simulink model "BMS_V4"  (R2017b)
settings: Solver=FixedStepDiscrete  StartTime=0.0  StopTime=inf  FixedStep=BASETIME  RelTol=1e-3  EnableMultiTasking=on
values from neighbouring files (symbols this model uses):
  AKT_BALANCE = uint16(8)    [BMS_V4_config.m]
  BALANCE = uint16(4)    [BMS_V4_config.m]
  BALANCE_RESISTOR = int32(5)    [BMS_V4_config.m]
  BALANCE_VEC = uint16(8)    [BMS_V4_config.m]
  CELL_SOC = uint16(7)    [BMS_V4_config.m]
  CELL_STATE = uint16(3)    [BMS_V4_config.m]
  CELL_TEMPERATURE = uint16(6)    [BMS_V4_config.m]
  CELL_VOLTAGE = uint16(5)    [BMS_V4_config.m]
  CELLACTBITFIELD = hex2dec('300')    [BMS_V4_config.m]
  CELLDEACTBITFIELD = hex2dec('100')    [BMS_V4_config.m]
  CELLT_BURST = uint16(6)    [BMS_V4_config.m]
  CELLV_BURST = uint16(5)    [BMS_V4_config.m]
  CLK_CYC_timer_1 = 586    [BMS_V4_config.m]
  CLK_CYC_timer_2 = 5860    [BMS_V4_config.m]
  CLK_CYC_timer_3 = 280    [BMS_V4_config.m]
  CLK_CYC_timer_4 = 586*100    (= 58600)    [BMS_V4_config.m]
  CLK_CYC_timer_5 = 5800*2    (= 11600)    [BMS_V4_config.m]
  CLK_CYC_timer_6 = 320    [BMS_V4_config.m]
  CN_CELLS = int32(40*3600)    [BMS_V4_config.m]
  CONTACTOR = uint16(1)    [BMS_V4_config.m]
  CONTACTOR_LOCKED = uint16(0)    [BMS_V4_config.m]
  CONTACTOR_UNLOCKED = uint16(1)    [BMS_V4_config.m]
  DEBUG_SEND_STATES = uint16(hex2dec('01'))    [BMS_V4_config.m]
  DELTA_SOC_BALANCE = int32(5*1e6)    [BMS_V4_config.m]
  DELTA_SOC_BALANCE_OFF = int32(1*1e5)    [BMS_V4_config.m]
  DETERMINE_MODEL_PARAMETER_ACT = uint16(100)    [BMS_V4_config.m]
  DETERMINE_MODEL_PARAMETER_SCC = uint16(101)    [BMS_V4_config.m]
  ERROR = uint16(1)    [BMS_V4_config.m]
  EXTERN_SIGNALS = uint16(1)    [BMS_V4_config.m]
  FREQUENCY_STEPS = uint16([25 50 75 100 150 250 500 750                                      1000 1500 2500 5000 7500                                      10010 10015 10025 10050 10075                                      10100 10150 10250 10500 10750                                      11000 11500])    [BMS_V4_config.m]
  GET_IMAG_PART_MFC = uint16(9)    [BMS_V4_config.m]
  GET_IMAG_PART_MSF = uint16(4)    [BMS_V4_config.m]
  GET_REAL_PART_MFC = uint16(8)    [BMS_V4_config.m]
  GET_REAL_PART_MSF = uint16(3)    [BMS_V4_config.m]
  IMU = uint16(7)    [BMS_V4_config.m]
  IMU_AMP_OFF = uint16(5)    [BMS_V4_config.m]
  IMU_DATA_READ_LOCUS_ACT = uint16(6)    [BMS_V4_config.m]
  IMU_DATA_READ_LOCUS_SCC = uint16(7)    [BMS_V4_config.m]
  IMU_DEBUG = uint16(9)    [BMS_V4_config.m]
  IMU_GET_DATA_MFC = uint16(8)    [BMS_V4_config.m]
  IMU_GET_DATA_MSF = uint16(3)    [BMS_V4_config.m]
  IMU_OFFSET_POLLING = uint16(11)    [BMS_V4_config.m]
  IMU_POLLING = uint16(2)    [BMS_V4_config.m]
  IMU_POWER = uint16(10)    [BMS_V4_config.m]
  IMU_SEND_IMAG = uint16(11)    [BMS_V4_config.m]
  IMU_SEND_REAL = uint16(10)    [BMS_V4_config.m]
  INDEX_IMAGPART = uint16(2)    [BMS_V4_config.m]
  INDEX_REALPART = uint16(1)    [BMS_V4_config.m]
  INFO = uint16(2)    [BMS_V4_config.m]
  INIT_OFFSET_AMPLITUDE = uint16(2)    [BMS_V4_config.m]
  LINE_CURRENT = uint16(3)    [BMS_V4_config.m]
  LINE_CURRENT_CANA = uint16(4)    [BMS_V4_config.m]
  LINE_CURRENT_SWITCH_THRESHOLD = int32(2*1e6)    [BMS_V4_config.m]
  NUM_OF_CELLS = uint16(16)    [BMS_V4_config.m]
  NUM_OF_FREQUENCIES_PSO = uint16(14)    [BMS_V4_config.m]
  NUM_OF_LINES = uint16(1)    [BMS_V4_config.m]
  NUM_OF_PARAMETER = single(5)    [BMS_V4_config.m]
  NUM_OF_SOC_POINTS = uint16(110)    [BMS_V4_config.m]
  P_L_BOUND = single([0.05;0.01;0.1;0.01;0.1])    [BMS_V4_config.m]
  P_U_BOUND = single([0.50;0.20;0.9;0.06;60])    [BMS_V4_config.m]
  PARA_ACT_SEND = uint16(101)    [BMS_V4_config.m]
  PARA_DATA_STORE_ACT = uint16(8)    [BMS_V4_config.m]
  PARA_DATA_STORE_SCC = uint16(9)    [BMS_V4_config.m]
  PARA_SCC_SEND = uint16(102)    [BMS_V4_config.m]
  PARTICLE_INIT = single(create_startparticle(P_L_BOUND,P_U_BOUND,NUM_OF_PARTICLE))    [BMS_V4_config.m]
  POLACT = hex2dec('00000BFF')    [BMS_V4_config.m]
  POLDEACT = hex2dec('000008FF')    [BMS_V4_config.m]
  PSO_PARA_DEBUG = uint16(13)    [BMS_V4_config.m]
  REQUEST_SOC_REF = uint16(1000)    [BMS_V4_config.m]
  SCALE_FACTOR_CH1 = single(0.66666666)    [BMS_V4_config.m]
  SCALE_FACTOR_CH2 = single(0.66666666)    [BMS_V4_config.m]
  SEND_CELL_SOC_ABS = uint16(199)    [BMS_V4_config.m]
  SHUT_DOWN_BALANCE_OFF = uint16(3)    [BMS_V4_config.m]
  SHUT_DOWN_BALANCE_ON = uint16(2)    [BMS_V4_config.m]
  START_IMU_MSL = uint16(3)    [BMS_V4_config.m]
  START_IMU_SCC = uint16(1)    [BMS_V4_config.m]
  SWITCH_IMU_OFF = uint16(2)    [BMS_V4_config.m]
  SWITCH_IMU_ON = uint16(1)    [BMS_V4_config.m]
  SWITCH_IMU_ON_OFF = uint16(4)    [BMS_V4_config.m]
  SYSTEM_DEBUG = uint16(12)    [BMS_V4_config.m]
  TIMEOUT_CANA = uint32(5000)    [BMS_V4_config.m]
  TIMEOUT_GATEWAY = uint32(500)    [BMS_V4_config.m]
  TS_SOC = single(0.010)    [BMS_V4_config.m]
  WARNING = uint16(2)    [BMS_V4_config.m]
libraries: c280xlib x44, c2833xlib x5, simulink x2, c2000lib x1, idelinklib_common x1
(part 2 of 8)

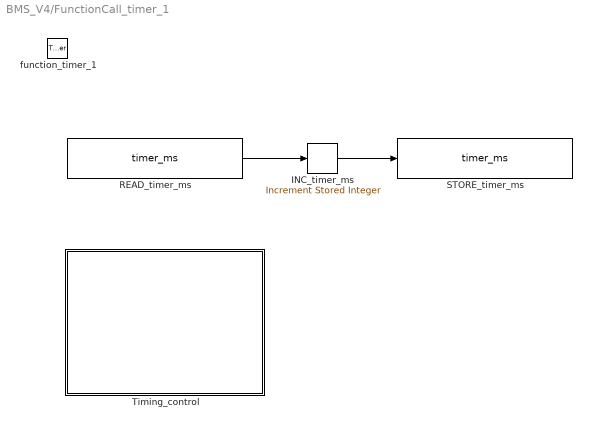
== system BMS_V4/FunctionCall_timer_1 ==
  function_timer_1 : TriggerPort  TriggerType=function-call  VariantControl=Variant
  INC_timer_ms : simulink/Additional Math & Discrete/Additional Math: Increment - Decrement/Increment Stored Integer
      settings: SourceProductName=Simulink
  READ_timer_ms : DataStoreRead  DataStoreName=timer_ms
  STORE_timer_ms : DataStoreWrite  DataStoreName=timer_ms
  Timing_control : Stateflow chart  TreatAsAtomicUnit=on
      settings: RTWSystemCode=Nonreusable function  RTWFcnNameOpts=Use subsystem name  RTWFileNameOpts=Use subsystem name
  wires:
  READ_timer_ms/1 -> INC_timer_ms/1
  INC_timer_ms/1 -> STORE_timer_ms/1

== system BMS_V4/FunctionCall_timer_2 ==
  function_timer_2 : TriggerPort  TriggerType=function-call  VariantControl=Variant
  calculation_soc_CC : MATLAB Function  TreatAsAtomicUnit=on
      settings: RTWSystemCode=Nonreusable function  RTWFcnNameOpts=Use subsystem name  RTWFileNameOpts=Use subsystem name  FunctionInterfaceSpec=Allow arguments

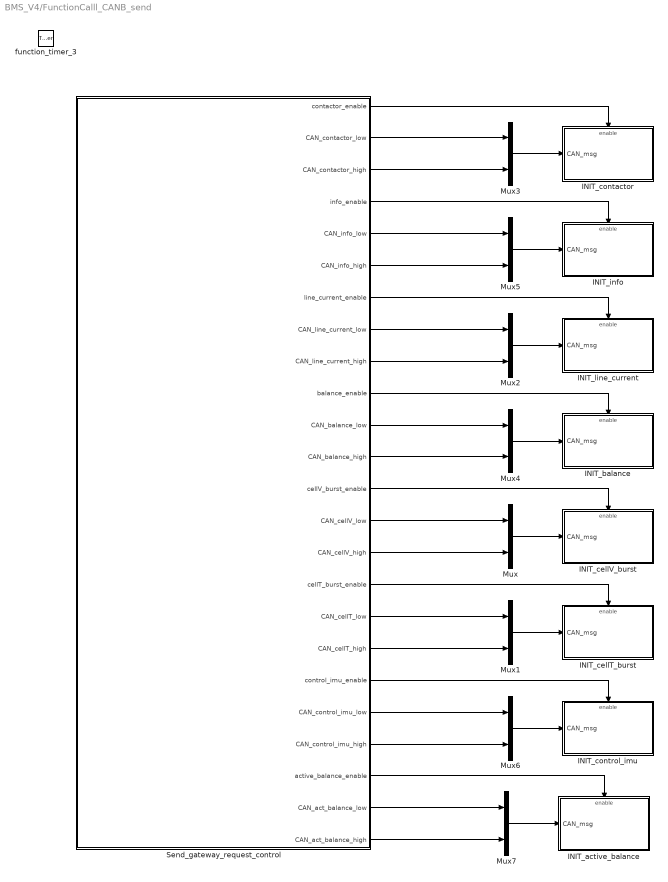
== system BMS_V4/FunctionCalll_CANB_send ==
  function_timer_3 : TriggerPort  TriggerType=function-call  VariantControl=Variant
  INIT_active_balance : Subsystem  TreatAsAtomicUnit=on
      settings: RTWSystemCode=Nonreusable function  RTWFcnNameOpts=Use subsystem name  RTWFileNameOpts=Use subsystem name
  INIT_balance : Subsystem  TreatAsAtomicUnit=on
      settings: RTWSystemCode=Nonreusable function  RTWFcnNameOpts=Use subsystem name  RTWFileNameOpts=Use subsystem name
  INIT_cellT_burst : Subsystem  TreatAsAtomicUnit=on
      settings: RTWSystemCode=Nonreusable function  RTWFcnNameOpts=Use subsystem name  RTWFileNameOpts=Use subsystem name
  INIT_cellV_burst : Subsystem  TreatAsAtomicUnit=on
      settings: RTWSystemCode=Nonreusable function  RTWFcnNameOpts=Use subsystem name  RTWFileNameOpts=Use subsystem name
  INIT_contactor : Subsystem  TreatAsAtomicUnit=on
      settings: RTWSystemCode=Nonreusable function  RTWFcnNameOpts=Use subsystem name  RTWFileNameOpts=Use subsystem name
  INIT_control_imu : Subsystem  TreatAsAtomicUnit=on
      settings: RTWSystemCode=Nonreusable function  RTWFcnNameOpts=Use subsystem name  RTWFileNameOpts=Use subsystem name
  INIT_info : Subsystem  TreatAsAtomicUnit=on
      settings: RTWSystemCode=Nonreusable function  RTWFcnNameOpts=Use subsystem name  RTWFileNameOpts=Use subsystem name
  INIT_line_current : Subsystem  TreatAsAtomicUnit=on
      settings: RTWSystemCode=Nonreusable function  RTWFcnNameOpts=Use subsystem name  RTWFileNameOpts=Use subsystem name
  Mux{,1..7} (8 alike) : Mux  Inputs=2
  Send_gateway_request_control : MATLAB Function  TreatAsAtomicUnit=on
      settings: RTWSystemCode=Nonreusable function  RTWFcnNameOpts=Use subsystem name  RTWFileNameOpts=Use subsystem name
  wires:
  Mux/1 -> INIT_cellV_burst/1(CAN_msg)
  Mux1/1 -> INIT_cellT_burst/1(CAN_msg)
  Mux2/1 -> INIT_line_current/1(CAN_msg)
  Mux3/1 -> INIT_contactor/1(CAN_msg)
  Mux4/1 -> INIT_balance/1(CAN_msg)
  Mux5/1 -> INIT_info/1(CAN_msg)
  Send_gateway_request_control/1(contactor_enable) -> INIT_contactor/Enable
  Send_gateway_request_control/2(CAN_contactor_low) -> Mux3/1
  Send_gateway_request_control/3(CAN_contactor_high) -> Mux3/2
  Send_gateway_request_control/5(CAN_info_low) -> Mux5/1
  Send_gateway_request_control/6(CAN_info_high) -> Mux5/2
  Send_gateway_request_control/4(info_enable) -> INIT_info/Enable
  Send_gateway_request_control/8(CAN_line_current_low) -> Mux2/1
  Send_gateway_request_control/9(CAN_line_current_high) -> Mux2/2
  Send_gateway_request_control/7(line_current_enable) -> INIT_line_current/Enable
  Send_gateway_request_control/10(balance_enable) -> INIT_balance/Enable
  Send_gateway_request_control/11(CAN_balance_low) -> Mux4/1
  Send_gateway_request_control/12(CAN_balance_high) -> Mux4/2
  Send_gateway_request_control/13(cellV_burst_enable) -> INIT_cellV_burst/Enable
  Send_gateway_request_control/14(CAN_cellV_low) -> Mux/1
  Send_gateway_request_control/15(CAN_cellV_high) -> Mux/2
  Send_gateway_request_control/17(CAN_cellT_low) -> Mux1/1
  Send_gateway_request_control/18(CAN_cellT_high) -> Mux1/2
  Send_gateway_request_control/16(cellT_burst_enable) -> INIT_cellT_burst/Enable
  Mux6/1 -> INIT_control_imu/1(CAN_msg)
  Send_gateway_request_control/19(control_imu_enable) -> INIT_control_imu/Enable
  Send_gateway_request_control/20(CAN_control_imu_low) -> Mux6/1
  Send_gateway_request_control/21(CAN_control_imu_high) -> Mux6/2
  Mux7/1 -> INIT_active_balance/1(CAN_msg)
  Send_gateway_request_control/22(active_balance_enable) -> INIT_active_balance/Enable
  Send_gateway_request_control/23(CAN_act_balance_low) -> Mux7/1
  Send_gateway_request_control/24(CAN_act_balance_high) -> Mux7/2

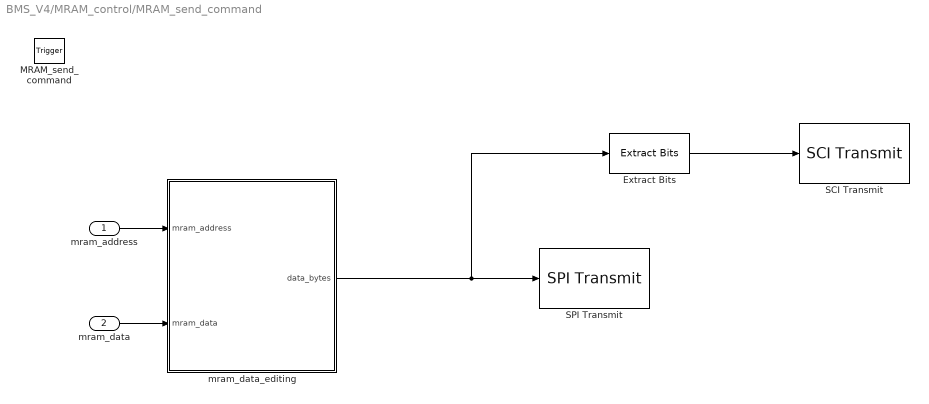
== system BMS_V4/MRAM_control/MRAM_send_command ==
  mram_address : Inport  OutDataTypeStr=uint32
  mram_data : Inport  Port=2  OutDataTypeStr=uint32
  MRAM_send_command : TriggerPort  TriggerType=function-call  VariantControl=Variant
      settings: CopyFcn=Stateflow.SLINSF.SimulinkMan.removeBlockPreDeleteFcn  PreDeleteFcn=Stateflow.SLINSF.SimulinkMan.unsafePredeleteFcn
  Extract Bits : simulink/Logic and Bit Operations/Extract Bits  bitsToExtract=Range ending with least significant bit  numBits=8  bitIdxRange=[0 7]  outScalingMode=Preserve fixed-point scaling
      settings: SourceProductName=Simulink
  SCI Transmit : c280xlib/SCI Transmit  sciModule=B  dataHead=''  dataTail=''  postInterrupt=off  numFifo=1
      settings: SourceProductName=Embedded Coder Support Package for Texas Instruments C2000 Processors
  SPI Transmit : c280xlib/SPI Transmit  SPISelect=SPI_A  ClockPolarity=Falling_edge  ClockPhase=No_delay  SPIModule=uint32(0)  Mode=Master  BusSpeed=uint32(1000000)  FirstBitToTransfer=Most significant bit (MSB)  ClockMode=0  BlockFunction=Write  RegisterAddress=0  OutputDataType=int8  OutputDataLength=1  BlockingMode=off  DataBits=8  UseCustomSSPin=Provided by the SPI peripheral  ActiveLowSSPin=Active low  Pin=0
      settings: SourceProductName=Embedded Coder Support Package for Texas Instruments C2000 Processors  SourceProductBaseCode=TIC2000
  mram_data_editing : MATLAB Function  TreatAsAtomicUnit=on
  wires:
  mram_address/1 -> mram_data_editing/1(mram_address)
  mram_data/1 -> mram_data_editing/2(mram_data)
  mram_data_editing/1(data_bytes) -> Extract Bits/1, SPI Transmit/1
  Extract Bits/1 -> SCI Transmit/1

== system BMS_V4/PARAMETER_ESTIMATION_control/send_ms_uart ==
  f : TriggerPort  TriggerType=function-call  VariantControl=Variant
      settings: CopyFcn=Stateflow.SLINSF.SimulinkMan.removeBlockPreDeleteFcn  PreDeleteFcn=Stateflow.SLINSF.SimulinkMan.unsafePredeleteFcn
  Data Store Read : DataStoreRead  Commented=on  DataStoreName=timer_ms
  SCI Transmit : c280xlib/SCI Transmit  Commented=on  sciModule=B  dataHead='S'  dataTail='E'  postInterrupt=off  numFifo=1
      settings: SourceProductName=Embedded Coder Support Package for Texas Instruments C2000 Processors
  wires:
  Data Store Read/1 -> SCI Transmit/1

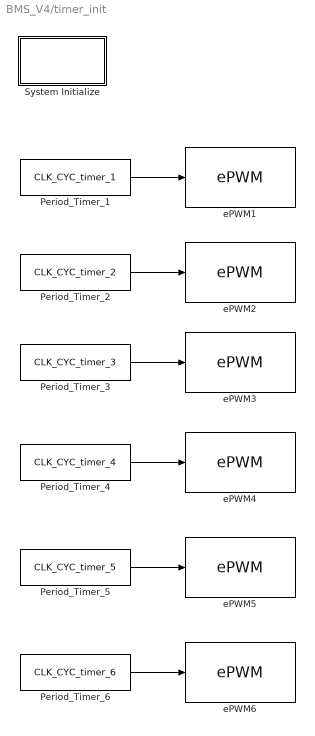
== system BMS_V4/timer_init ==
  Period_Timer_1 : Constant  Value=CLK_CYC_timer_1
  Period_Timer_2 : Constant  Value=CLK_CYC_timer_2
  Period_Timer_3 : Constant  Value=CLK_CYC_timer_3
  Period_Timer_4 : Constant  Value=CLK_CYC_timer_4
  Period_Timer_5 : Constant  Value=CLK_CYC_timer_5
  Period_Timer_6 : Constant  Value=CLK_CYC_timer_6
  System Initialize : Subsystem  mask(System Initialize){ShowInLibBrowser=0}
      mask prompts: ShowInLibBrowser "Simulink:masks:CustCodeMaskParam1_MP"
      settings: CopyFcn=cccopyfcn(gcb)  OpenFcn=ccopenfcn('System Initialize Function')
      mask Help: eval('feval(''rtwprivate'',''rtwhelpview'',''rtw_sys_initialize_block'')');
      mask Display: disp('System\nInitialize');
  ePWM1 : c280xlib/ePWM  checkMode=off  useModule=ePWM1  periodUnits=Clock cycles  timerSource=Input port  timerPeriod_clk=64000  timerPeriod_sec=0.0001  tbshadow=Counter equals to zero  countingMode=Up  phaseActiveEnable=Disable  phaseDirection=Count down after sync  phaseActive=0  synchronizationEnable=off  synchronizationOption=Disable  clockPrescale=128  HSclockPrescale=2  ePWMxAStatus=off  CMPAUnits=Clock cycles  CMPASource=Specify via dialog  CMPAValue_per=50  CMPAValue_clk=32000  enCMPAshadow=Counter equals to zero  ePWMxAactionLogic1=Do nothing  ePWMxAactionLogic2=Clear  ePWMxAactionLogic3=Set  ePWMxAactionLogic4=Do nothing  ePWMxAactionLogic5=Do nothing  ePWMxAactionLogic6=Do nothing  ePWMxALoadMode=Load on counter equals to zero (CTR=Zero)  ePWMxACSFenable=off  ePWMxACSFvalue=Forcing disable  ePWMxASFreload=Zero  enHRPWM=off  HRPWM_LoadMode=Counter equals to zero (CTR=ZERO)  HRPWM_CTLMode=Phase control mode  HRPWM_EDGMode=Both edge  enSFO=on  ePWMxBStatus=off  CMPBUnits=Clock cycles  CMPBSource=Specify via dialog  CMPBValue_per=50  CMPBValue_clk=32000  enCMPBshadow=Counter equals to zero  ePWMxBactionLogic1=Do nothing  ePWMxBactionLogic2=Set  ePWMxBactionLogic3=Do nothing  ePWMxBactionLogic4=Do nothing  ePWMxBactionLogic5=Clear  ePWMxBactionLogic6=Do nothing  ePWMxBLoadMode=Load on counter equals to zero (CTR=Zero)  ePWMxBCSFenable=off  ePWMxBCSFvalue=Forcing disable  ePWMxBSFreload=Zero  enableDBePWMxA=off  enableDBePWMxB=off  DBpolarity=Active high (AH)  DBedgeDelay=Positive  DBSource_ePWMxA=ePWMxA  DBSource_ePWMxB=ePWMxA  DBperiodSource=Specify via dialog  REDperiod=0  FEDperiod=0  adcstartModuleA=off  adcrequestEventA=First event  adcstartEventA=Counter equals to zero (CTR=Zero)  adcstartModuleB=off  adcrequestEventB=First event  adcstartEventB=Counter equals to zero (CTR=Zero)  intEn=off  intPrd=First event  intSel=Counter equals to zero (CTR=Zero)  chopperEnable=off  chopperFrequency=1  chopperFirstwidth=1  chopperDuty=12.5%  tripZonesource=Specify via dialog  tzselOSHT1=off  tzselOSHT2=off  tzselOSHT3=off  tzselOSHT4=off  tzselOSHT5=off  tzselOSHT6=off  tzselCBC1=off  tzselCBC2=off  tzselCBC3=off  tzselCBC4=off  tzselCBC5=off  tzselCBC6=off  enTzOstIntr=off  enTzCbcIntr=off  ePWMxAforced=No action  ePWMxBforced=No action  timerPeriod=-1  ePWMxAValue=0  ePWMxBValue=0  tripZoneoption=One-shot trip (OSHT)
      settings: SourceProductName=Embedded Coder Support Package for Texas Instruments C2000 Processors  SourceProductBaseCode=TIC2000
  ePWM2 : c280xlib/ePWM  checkMode=off  useModule=ePWM2  periodUnits=Clock cycles  timerSource=Input port  timerPeriod_clk=64000  timerPeriod_sec=0.0001  tbshadow=Counter equals to zero  countingMode=Up  phaseActiveEnable=Disable  phaseDirection=Count down after sync  phaseActive=0  synchronizationEnable=off  synchronizationOption=Disable  clockPrescale=128  HSclockPrescale=2  ePWMxAStatus=off  CMPAUnits=Clock cycles  CMPASource=Specify via dialog  CMPAValue_per=50  CMPAValue_clk=32000  enCMPAshadow=Counter equals to zero  ePWMxAactionLogic1=Do nothing  ePWMxAactionLogic2=Clear  ePWMxAactionLogic3=Set  ePWMxAactionLogic4=Do nothing  ePWMxAactionLogic5=Do nothing  ePWMxAactionLogic6=Do nothing  ePWMxALoadMode=Load on counter equals to zero (CTR=Zero)  ePWMxACSFenable=off  ePWMxACSFvalue=Forcing disable  ePWMxASFreload=Zero  enHRPWM=off  HRPWM_LoadMode=Counter equals to zero (CTR=ZERO)  HRPWM_CTLMode=Phase control mode  HRPWM_EDGMode=Both edge  enSFO=on  ePWMxBStatus=off  CMPBUnits=Clock cycles  CMPBSource=Specify via dialog  CMPBValue_per=50  CMPBValue_clk=32000  enCMPBshadow=Counter equals to zero  ePWMxBactionLogic1=Do nothing  ePWMxBactionLogic2=Set  ePWMxBactionLogic3=Do nothing  ePWMxBactionLogic4=Do nothing  ePWMxBactionLogic5=Clear  ePWMxBactionLogic6=Do nothing  ePWMxBLoadMode=Load on counter equals to zero (CTR=Zero)  ePWMxBCSFenable=off  ePWMxBCSFvalue=Forcing disable  ePWMxBSFreload=Zero  enableDBePWMxA=off  enableDBePWMxB=off  DBpolarity=Active high (AH)  DBedgeDelay=Positive  DBSource_ePWMxA=ePWMxA  DBSource_ePWMxB=ePWMxA  DBperiodSource=Specify via dialog  REDperiod=0  FEDperiod=0  adcstartModuleA=off  adcrequestEventA=First event  adcstartEventA=Counter equals to zero (CTR=Zero)  adcstartModuleB=off  adcrequestEventB=First event  adcstartEventB=Counter equals to zero (CTR=Zero)  intEn=off  intPrd=First event  intSel=Counter equals to zero (CTR=Zero)  chopperEnable=off  chopperFrequency=1  chopperFirstwidth=1  chopperDuty=12.5%  tripZonesource=Specify via dialog  tzselOSHT1=off  tzselOSHT2=off  tzselOSHT3=off  tzselOSHT4=off  tzselOSHT5=off  tzselOSHT6=off  tzselCBC1=off  tzselCBC2=off  tzselCBC3=off  tzselCBC4=off  tzselCBC5=off  tzselCBC6=off  enTzOstIntr=off  enTzCbcIntr=off  ePWMxAforced=No action  ePWMxBforced=No action  timerPeriod=-1  ePWMxAValue=0  ePWMxBValue=0  tripZoneoption=One-shot trip (OSHT)
      settings: SourceProductName=Embedded Coder Support Package for Texas Instruments C2000 Processors  SourceProductBaseCode=TIC2000
  ePWM3 : c280xlib/ePWM  checkMode=off  useModule=ePWM3  periodUnits=Clock cycles  timerSource=Input port  timerPeriod_clk=64000  timerPeriod_sec=0.0001  tbshadow=Counter equals to zero  countingMode=Up  phaseActiveEnable=Disable  phaseDirection=Count down after sync  phaseActive=0  synchronizationEnable=off  synchronizationOption=Disable  clockPrescale=128  HSclockPrescale=2  ePWMxAStatus=off  CMPAUnits=Clock cycles  CMPASource=Specify via dialog  CMPAValue_per=50  CMPAValue_clk=32000  enCMPAshadow=Counter equals to zero  ePWMxAactionLogic1=Do nothing  ePWMxAactionLogic2=Clear  ePWMxAactionLogic3=Set  ePWMxAactionLogic4=Do nothing  ePWMxAactionLogic5=Do nothing  ePWMxAactionLogic6=Do nothing  ePWMxALoadMode=Load on counter equals to zero (CTR=Zero)  ePWMxACSFenable=off  ePWMxACSFvalue=Forcing disable  ePWMxASFreload=Zero  enHRPWM=off  HRPWM_LoadMode=Counter equals to zero (CTR=ZERO)  HRPWM_CTLMode=Phase control mode  HRPWM_EDGMode=Both edge  enSFO=on  ePWMxBStatus=off  CMPBUnits=Clock cycles  CMPBSource=Specify via dialog  CMPBValue_per=50  CMPBValue_clk=32000  enCMPBshadow=Counter equals to zero  ePWMxBactionLogic1=Do nothing  ePWMxBactionLogic2=Set  ePWMxBactionLogic3=Do nothing  ePWMxBactionLogic4=Do nothing  ePWMxBactionLogic5=Clear  ePWMxBactionLogic6=Do nothing  ePWMxBLoadMode=Load on counter equals to zero (CTR=Zero)  ePWMxBCSFenable=off  ePWMxBCSFvalue=Forcing disable  ePWMxBSFreload=Zero  enableDBePWMxA=off  enableDBePWMxB=off  DBpolarity=Active high (AH)  DBedgeDelay=Positive  DBSource_ePWMxA=ePWMxA  DBSource_ePWMxB=ePWMxA  DBperiodSource=Specify via dialog  REDperiod=0  FEDperiod=0  adcstartModuleA=off  adcrequestEventA=First event  adcstartEventA=Counter equals to zero (CTR=Zero)  adcstartModuleB=off  adcrequestEventB=First event  adcstartEventB=Counter equals to zero (CTR=Zero)  intEn=off  intPrd=First event  intSel=Counter equals to zero (CTR=Zero)  chopperEnable=off  chopperFrequency=1  chopperFirstwidth=1  chopperDuty=12.5%  tripZonesource=Specify via dialog  tzselOSHT1=off  tzselOSHT2=off  tzselOSHT3=off  tzselOSHT4=off  tzselOSHT5=off  tzselOSHT6=off  tzselCBC1=off  tzselCBC2=off  tzselCBC3=off  tzselCBC4=off  tzselCBC5=off  tzselCBC6=off  enTzOstIntr=off  enTzCbcIntr=off  ePWMxAforced=No action  ePWMxBforced=No action  timerPeriod=-1  ePWMxAValue=0  ePWMxBValue=0  tripZoneoption=One-shot trip (OSHT)
      settings: SourceProductName=Embedded Coder Support Package for Texas Instruments C2000 Processors  SourceProductBaseCode=TIC2000
  ePWM4 : c280xlib/ePWM  checkMode=off  useModule=ePWM4  periodUnits=Clock cycles  timerSource=Input port  timerPeriod_clk=64000  timerPeriod_sec=0.0001  tbshadow=Counter equals to zero  countingMode=Up  phaseActiveEnable=Disable  phaseDirection=Count down after sync  phaseActive=0  synchronizationEnable=off  synchronizationOption=Disable  clockPrescale=128  HSclockPrescale=2  ePWMxAStatus=off  CMPAUnits=Clock cycles  CMPASource=Specify via dialog  CMPAValue_per=50  CMPAValue_clk=32000  enCMPAshadow=Counter equals to zero  ePWMxAactionLogic1=Do nothing  ePWMxAactionLogic2=Clear  ePWMxAactionLogic3=Set  ePWMxAactionLogic4=Do nothing  ePWMxAactionLogic5=Do nothing  ePWMxAactionLogic6=Do nothing  ePWMxALoadMode=Load on counter equals to zero (CTR=Zero)  ePWMxACSFenable=off  ePWMxACSFvalue=Forcing disable  ePWMxASFreload=Zero  enHRPWM=off  HRPWM_LoadMode=Counter equals to zero (CTR=ZERO)  HRPWM_CTLMode=Phase control mode  HRPWM_EDGMode=Both edge  enSFO=on  ePWMxBStatus=off  CMPBUnits=Clock cycles  CMPBSource=Specify via dialog  CMPBValue_per=50  CMPBValue_clk=32000  enCMPBshadow=Counter equals to zero  ePWMxBactionLogic1=Do nothing  ePWMxBactionLogic2=Set  ePWMxBactionLogic3=Do nothing  ePWMxBactionLogic4=Do nothing  ePWMxBactionLogic5=Clear  ePWMxBactionLogic6=Do nothing  ePWMxBLoadMode=Load on counter equals to zero (CTR=Zero)  ePWMxBCSFenable=off  ePWMxBCSFvalue=Forcing disable  ePWMxBSFreload=Zero  enableDBePWMxA=off  enableDBePWMxB=off  DBpolarity=Active high (AH)  DBedgeDelay=Positive  DBSource_ePWMxA=ePWMxA  DBSource_ePWMxB=ePWMxA  DBperiodSource=Specify via dialog  REDperiod=0  FEDperiod=0  adcstartModuleA=off  adcrequestEventA=First event  adcstartEventA=Counter equals to zero (CTR=Zero)  adcstartModuleB=off  adcrequestEventB=First event  adcstartEventB=Counter equals to zero (CTR=Zero)  intEn=off  intPrd=First event  intSel=Counter equals to zero (CTR=Zero)  chopperEnable=off  chopperFrequency=1  chopperFirstwidth=1  chopperDuty=12.5%  tripZonesource=Specify via dialog  tzselOSHT1=off  tzselOSHT2=off  tzselOSHT3=off  tzselOSHT4=off  tzselOSHT5=off  tzselOSHT6=off  tzselCBC1=off  tzselCBC2=off  tzselCBC3=off  tzselCBC4=off  tzselCBC5=off  tzselCBC6=off  enTzOstIntr=off  enTzCbcIntr=off  ePWMxAforced=No action  ePWMxBforced=No action  timerPeriod=-1  ePWMxAValue=0  ePWMxBValue=0  tripZoneoption=One-shot trip (OSHT)
      settings: SourceProductName=Embedded Coder Support Package for Texas Instruments C2000 Processors  SourceProductBaseCode=TIC2000
  ePWM5 : c280xlib/ePWM  checkMode=off  useModule=ePWM5  periodUnits=Clock cycles  timerSource=Input port  timerPeriod_clk=64000  timerPeriod_sec=0.0001  tbshadow=Counter equals to zero  countingMode=Up  phaseActiveEnable=Disable  phaseDirection=Count down after sync  phaseActive=0  synchronizationEnable=off  synchronizationOption=Disable  clockPrescale=128  HSclockPrescale=2  ePWMxAStatus=off  CMPAUnits=Clock cycles  CMPASource=Specify via dialog  CMPAValue_per=50  CMPAValue_clk=32000  enCMPAshadow=Counter equals to zero  ePWMxAactionLogic1=Do nothing  ePWMxAactionLogic2=Clear  ePWMxAactionLogic3=Set  ePWMxAactionLogic4=Do nothing  ePWMxAactionLogic5=Do nothing  ePWMxAactionLogic6=Do nothing  ePWMxALoadMode=Load on counter equals to zero (CTR=Zero)  ePWMxACSFenable=off  ePWMxACSFvalue=Forcing disable  ePWMxASFreload=Zero  enHRPWM=off  HRPWM_LoadMode=Counter equals to zero (CTR=ZERO)  HRPWM_CTLMode=Phase control mode  HRPWM_EDGMode=Both edge  enSFO=on  ePWMxBStatus=off  CMPBUnits=Clock cycles  CMPBSource=Specify via dialog  CMPBValue_per=50  CMPBValue_clk=32000  enCMPBshadow=Counter equals to zero  ePWMxBactionLogic1=Do nothing  ePWMxBactionLogic2=Set  ePWMxBactionLogic3=Do nothing  ePWMxBactionLogic4=Do nothing  ePWMxBactionLogic5=Clear  ePWMxBactionLogic6=Do nothing  ePWMxBLoadMode=Load on counter equals to zero (CTR=Zero)  ePWMxBCSFenable=off  ePWMxBCSFvalue=Forcing disable  ePWMxBSFreload=Zero  enableDBePWMxA=off  enableDBePWMxB=off  DBpolarity=Active high (AH)  DBedgeDelay=Positive  DBSource_ePWMxA=ePWMxA  DBSource_ePWMxB=ePWMxA  DBperiodSource=Specify via dialog  REDperiod=0  FEDperiod=0  adcstartModuleA=off  adcrequestEventA=First event  adcstartEventA=Counter equals to zero (CTR=Zero)  adcstartModuleB=off  adcrequestEventB=First event  adcstartEventB=Counter equals to zero (CTR=Zero)  intEn=off  intPrd=First event  intSel=Counter equals to zero (CTR=Zero)  chopperEnable=off  chopperFrequency=1  chopperFirstwidth=1  chopperDuty=12.5%  tripZonesource=Specify via dialog  tzselOSHT1=off  tzselOSHT2=off  tzselOSHT3=off  tzselOSHT4=off  tzselOSHT5=off  tzselOSHT6=off  tzselCBC1=off  tzselCBC2=off  tzselCBC3=off  tzselCBC4=off  tzselCBC5=off  tzselCBC6=off  enTzOstIntr=off  enTzCbcIntr=off  ePWMxAforced=No action  ePWMxBforced=No action  timerPeriod=-1  ePWMxAValue=0  ePWMxBValue=0  tripZoneoption=One-shot trip (OSHT)
      settings: SourceProductName=Embedded Coder Support Package for Texas Instruments C2000 Processors  SourceProductBaseCode=TIC2000
  ePWM6 : c280xlib/ePWM  checkMode=off  useModule=ePWM6  periodUnits=Clock cycles  timerSource=Input port  timerPeriod_clk=64000  timerPeriod_sec=0.0001  tbshadow=Counter equals to zero  countingMode=Up  phaseActiveEnable=Disable  phaseDirection=Count down after sync  phaseActive=0  synchronizationEnable=off  synchronizationOption=Disable  clockPrescale=128  HSclockPrescale=2  ePWMxAStatus=off  CMPAUnits=Clock cycles  CMPASource=Specify via dialog  CMPAValue_per=50  CMPAValue_clk=32000  enCMPAshadow=Counter equals to zero  ePWMxAactionLogic1=Do nothing  ePWMxAactionLogic2=Clear  ePWMxAactionLogic3=Set  ePWMxAactionLogic4=Do nothing  ePWMxAactionLogic5=Do nothing  ePWMxAactionLogic6=Do nothing  ePWMxALoadMode=Load on counter equals to zero (CTR=Zero)  ePWMxACSFenable=off  ePWMxACSFvalue=Forcing disable  ePWMxASFreload=Zero  enHRPWM=off  HRPWM_LoadMode=Counter equals to zero (CTR=ZERO)  HRPWM_CTLMode=Phase control mode  HRPWM_EDGMode=Both edge  enSFO=on  ePWMxBStatus=off  CMPBUnits=Clock cycles  CMPBSource=Specify via dialog  CMPBValue_per=50  CMPBValue_clk=32000  enCMPBshadow=Counter equals to zero  ePWMxBactionLogic1=Do nothing  ePWMxBactionLogic2=Set  ePWMxBactionLogic3=Do nothing  ePWMxBactionLogic4=Do nothing  ePWMxBactionLogic5=Clear  ePWMxBactionLogic6=Do nothing  ePWMxBLoadMode=Load on counter equals to zero (CTR=Zero)  ePWMxBCSFenable=off  ePWMxBCSFvalue=Forcing disable  ePWMxBSFreload=Zero  enableDBePWMxA=off  enableDBePWMxB=off  DBpolarity=Active high (AH)  DBedgeDelay=Positive  DBSource_ePWMxA=ePWMxA  DBSource_ePWMxB=ePWMxA  DBperiodSource=Specify via dialog  REDperiod=0  FEDperiod=0  adcstartModuleA=off  adcrequestEventA=First event  adcstartEventA=Counter equals to zero (CTR=Zero)  adcstartModuleB=off  adcrequestEventB=First event  adcstartEventB=Counter equals to zero (CTR=Zero)  intEn=off  intPrd=First event  intSel=Counter equals to zero (CTR=Zero)  chopperEnable=off  chopperFrequency=1  chopperFirstwidth=1  chopperDuty=12.5%  tripZonesource=Specify via dialog  tzselOSHT1=off  tzselOSHT2=off  tzselOSHT3=off  tzselOSHT4=off  tzselOSHT5=off  tzselOSHT6=off  tzselCBC1=off  tzselCBC2=off  tzselCBC3=off  tzselCBC4=off  tzselCBC5=off  tzselCBC6=off  enTzOstIntr=off  enTzCbcIntr=off  ePWMxAforced=No action  ePWMxBforced=No action  timerPeriod=-1  ePWMxAValue=0  ePWMxBValue=0  tripZoneoption=One-shot trip (OSHT)
      settings: SourceProductName=Embedded Coder Support Package for Texas Instruments C2000 Processors  SourceProductBaseCode=TIC2000
  wires:
  Period_Timer_1/1 -> ePWM1/1
  Period_Timer_2/1 -> ePWM2/1
  Period_Timer_3/1 -> ePWM3/1
  Period_Timer_4/1 -> ePWM4/1
  Period_Timer_5/1 -> ePWM5/1
  Period_Timer_6/1 -> ePWM6/1

== system BMS_V4/FunctionCall_CANA_RX/handle_imu_debug ==
  CAN_msg : Inport
  handle_imu_debug : TriggerPort  TriggerType=function-call  VariantControl=Variant
  proceeding_imu_debug : MATLAB Function  TreatAsAtomicUnit=on
      settings: RTWSystemCode=Nonreusable function  RTWFcnNameOpts=Use subsystem name  RTWFileNameOpts=Use subsystem name
  wires:
  CAN_msg/1 -> proceeding_imu_debug/1(msg)

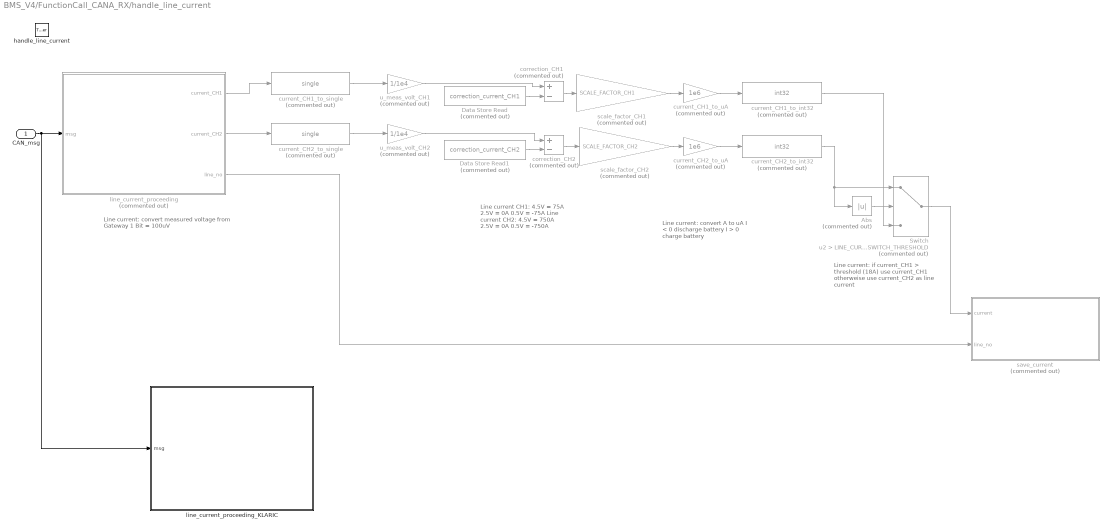
== system BMS_V4/FunctionCall_CANA_RX/handle_line_current ==
  note: Line current:
      | if current_CH1 > threshold (18A)
      | use current_CH1 otherweise
      | use current_CH2 as line current
  note: Line current:
      | convert A to uA
      | I < 0 discharge battery
      | I > 0 charge battery
  note: Line current CH1:
      | 4.5V = 75A
      | 2.5V = 0A
      | 0.5V = -75A
      | Line current CH2:
      | 4.5V = 750A
      | 2.5V = 0A
      | 0.5V = -750A
  note: Line current:
      | convert measured voltage from Gateway
      | 1 Bit = 100uV
  CAN_msg : Inport
  handle_line_current : TriggerPort  TriggerType=function-call  VariantControl=Variant
  Abs : Abs  Commented=on
  Data Store Read : DataStoreRead  Commented=on  DataStoreName=correction_current_CH1
  Data Store Read1 : DataStoreRead  Commented=on  DataStoreName=correction_current_CH2
  Switch : Switch  Commented=on  Criteria=u2 > Threshold  Threshold=LINE_CURRENT_SWITCH_THRESHOLD  OutDataTypeStr=int32
  correction_CH1 : Sum  Commented=on  Inputs=+-
  correction_CH2 : Sum  Commented=on  Inputs=+-
  current_CH1_to_int32 : DataTypeConversion  Commented=on  OutDataTypeStr=int32
  current_CH1_to_single : DataTypeConversion  Commented=on  OutDataTypeStr=single
  current_CH1_to_uA : Gain  Commented=on  Gain=1e6
  current_CH2_to_int32 : DataTypeConversion  Commented=on  OutDataTypeStr=int32
  current_CH2_to_single : DataTypeConversion  Commented=on  OutDataTypeStr=single
  current_CH2_to_uA : Gain  Commented=on  Gain=1e6
  line_current_proceeding : MATLAB Function  Commented=on  TreatAsAtomicUnit=on
      settings: RTWSystemCode=Nonreusable function  RTWFcnNameOpts=Use subsystem name  RTWFileNameOpts=Use subsystem name
  line_current_proceeding_KLARIC : MATLAB Function  TreatAsAtomicUnit=on
      settings: RTWSystemCode=Nonreusable function  RTWFcnNameOpts=Use subsystem name  RTWFileNameOpts=Use subsystem name
  save_current : MATLAB Function  Commented=on  TreatAsAtomicUnit=on
      settings: RTWSystemCode=Nonreusable function  RTWFcnNameOpts=Use subsystem name  RTWFileNameOpts=Use subsystem name
  scale_factor_CH1 : Gain  Commented=on  Gain=SCALE_FACTOR_CH1
  scale_factor_CH2 : Gain  Commented=on  Gain=SCALE_FACTOR_CH2
  u_meas_volt_CH1 : Gain  Commented=on  Gain=1/1e4
  u_meas_volt_CH2 : Gain  Commented=on  Gain=1/1e4
  wires:
  CAN_msg/1 -> line_current_proceeding/1(msg), line_current_proceeding_KLARIC/1(msg)
  line_current_proceeding/1(current_CH1) -> current_CH1_to_single/1
  current_CH1_to_uA/1 -> current_CH1_to_int32/1
  current_CH2_to_uA/1 -> current_CH2_to_int32/1
  Abs/1 -> Switch/2
  line_current_proceeding/3(line_no) -> save_current/2(line_no)
  line_current_proceeding/2(current_CH2) -> current_CH2_to_single/1
  u_meas_volt_CH1/1 -> correction_CH1/1
  correction_CH1/1 -> scale_factor_CH1/1
  Data Store Read/1 -> correction_CH1/2
  current_CH1_to_single/1 -> u_meas_volt_CH1/1
  scale_factor_CH1/1 -> current_CH1_to_uA/1
  current_CH2_to_single/1 -> u_meas_volt_CH2/1
  Data Store Read1/1 -> correction_CH2/2
  u_meas_volt_CH2/1 -> correction_CH2/1
  correction_CH2/1 -> scale_factor_CH2/1
  scale_factor_CH2/1 -> current_CH2_to_uA/1
  current_CH2_to_int32/1 -> Switch/1, Abs/1
  Switch/1 -> save_current/1(current)
  current_CH1_to_int32/1 -> Switch/3

== system BMS_V4/FunctionCall_CANA_RX/handle_pso_debug ==
  CAN_msg : Inport
  handle_system_debug : TriggerPort  TriggerType=function-call  VariantControl=Variant
  proceeding_pso_debug : MATLAB Function  TreatAsAtomicUnit=on
      settings: RTWSystemCode=Nonreusable function  RTWFcnNameOpts=Use subsystem name  RTWFileNameOpts=Use subsystem name
  wires:
  CAN_msg/1 -> proceeding_pso_debug/1(msg)

== system BMS_V4/FunctionCall_CANA_RX/handle_system_debug ==
  CAN_msg : Inport
  handle_system_debug : TriggerPort  TriggerType=function-call  VariantControl=Variant
  proceeding_system_debug : MATLAB Function  TreatAsAtomicUnit=on
      settings: RTWSystemCode=Nonreusable function  RTWFcnNameOpts=Use subsystem name  RTWFileNameOpts=Use subsystem name
  wires:
  CAN_msg/1 -> proceeding_system_debug/1(msg)

== system BMS_V4/FunctionCall_CANA_send/SEND_balance_vec ==
  CAN_msg : Inport
  Enable : EnablePort
  CAN_send_balance_vec : c280xlib/eCAN Transmit  chipFamily=C280x  useModule=eCAN_A  mailboxNo=22  messageID=ID_SEND_BALANCE_VEC  messageType=Standard (11-bit identifier)  enableBlockingMode=off  postInterrupt=off  interruptLine=0
      settings: SourceProductName=Embedded Coder Support Package for Texas Instruments C2000 Processors  SourceProductBaseCode=TIC2000
  wires:
  CAN_msg/1 -> CAN_send_balance_vec/1

== system BMS_V4/FunctionCall_CANA_send/SEND_cell_soc ==
  CAN_msg : Inport
  Enable : EnablePort
  CAN_send_cell_soc : c280xlib/eCAN Transmit  chipFamily=C280x  useModule=eCAN_A  mailboxNo=21  messageID=ID_SEND_CELL_SOC  messageType=Standard (11-bit identifier)  enableBlockingMode=off  postInterrupt=off  interruptLine=0
      settings: SourceProductName=Embedded Coder Support Package for Texas Instruments C2000 Processors  SourceProductBaseCode=TIC2000
  wires:
  CAN_msg/1 -> CAN_send_cell_soc/1

== system BMS_V4/FunctionCall_CANA_send/SEND_cell_states ==
  CAN_msg : Inport
  Enable : EnablePort
  CAN_send_cell_states : c280xlib/eCAN Transmit  chipFamily=C280x  useModule=eCAN_A  mailboxNo=17  messageID=ID_SEND_SYSTEM_STATES  messageType=Standard (11-bit identifier)  enableBlockingMode=off  postInterrupt=off  interruptLine=0
      settings: SourceProductName=Embedded Coder Support Package for Texas Instruments C2000 Processors  SourceProductBaseCode=TIC2000
  wires:
  CAN_msg/1 -> CAN_send_cell_states/1

== system BMS_V4/FunctionCall_CANA_send/SEND_cell_temperature ==
  CAN_msg : Inport
  Enable : EnablePort
  CAN_send_cell_temperature : c280xlib/eCAN Transmit  chipFamily=C280x  useModule=eCAN_A  mailboxNo=20  messageID=ID_SEND_CELL_TEMPERATURE  messageType=Standard (11-bit identifier)  enableBlockingMode=off  postInterrupt=off  interruptLine=0
      settings: SourceProductName=Embedded Coder Support Package for Texas Instruments C2000 Processors  SourceProductBaseCode=TIC2000
  wires:
  CAN_msg/1 -> CAN_send_cell_temperature/1

== system BMS_V4/FunctionCall_CANA_send/SEND_cell_voltage ==
  CAN_msg : Inport
  Enable : EnablePort
  CAN_send_cell_voltage : c280xlib/eCAN Transmit  chipFamily=C280x  useModule=eCAN_A  mailboxNo=19  messageID=ID_SEND_CELL_VOLTAGE  messageType=Standard (11-bit identifier)  enableBlockingMode=off  postInterrupt=off  interruptLine=0
      settings: SourceProductName=Embedded Coder Support Package for Texas Instruments C2000 Processors  SourceProductBaseCode=TIC2000
  wires:
  CAN_msg/1 -> CAN_send_cell_voltage/1

== system BMS_V4/FunctionCall_CANA_send/SEND_error ==
  CAN_msg : Inport
  Enable : EnablePort
  CAN_send_error : c280xlib/eCAN Transmit  chipFamily=C280x  useModule=eCAN_A  mailboxNo=16  messageID=ID_SEND_ERROR  messageType=Standard (11-bit identifier)  enableBlockingMode=off  postInterrupt=off  interruptLine=0
      settings: SourceProductName=Embedded Coder Support Package for Texas Instruments C2000 Processors  SourceProductBaseCode=TIC2000
  wires:
  CAN_msg/1 -> CAN_send_error/1

== system BMS_V4/FunctionCall_CANA_send/SEND_imu_debug ==
  CAN_msg : Inport
  Enable : EnablePort
  CAN_send_imu_debug : c280xlib/eCAN Transmit  chipFamily=C280x  useModule=eCAN_A  mailboxNo=24  messageID=ID_IMU_DEBUG  messageType=Standard (11-bit identifier)  enableBlockingMode=off  postInterrupt=off  interruptLine=0
      settings: SourceProductName=Embedded Coder Support Package for Texas Instruments C2000 Processors  SourceProductBaseCode=TIC2000
  wires:
  CAN_msg/1 -> CAN_send_imu_debug/1

== system BMS_V4/FunctionCall_CANA_send/SEND_imu_imagpart ==
  CAN_msg : Inport
  Enable : EnablePort
  CAN_send_imu_imagpart : c280xlib/eCAN Transmit  chipFamily=C280x  useModule=eCAN_A  mailboxNo=28  messageID=ID_IMU_IMAG  messageType=Standard (11-bit identifier)  enableBlockingMode=off  postInterrupt=off  interruptLine=0
      settings: SourceProductName=Embedded Coder Support Package for Texas Instruments C2000 Processors  SourceProductBaseCode=TIC2000
  wires:
  CAN_msg/1 -> CAN_send_imu_imagpart/1

== system BMS_V4/FunctionCall_CANA_send/SEND_imu_realpart ==
  CAN_msg : Inport
  Enable : EnablePort
  CAN_send_imu_realpart : c280xlib/eCAN Transmit  chipFamily=C280x  useModule=eCAN_A  mailboxNo=27  messageID=ID_IMU_REAL  messageType=Standard (11-bit identifier)  enableBlockingMode=off  postInterrupt=off  interruptLine=0
      settings: SourceProductName=Embedded Coder Support Package for Texas Instruments C2000 Processors  SourceProductBaseCode=TIC2000
  wires:
  CAN_msg/1 -> CAN_send_imu_realpart/1

== system BMS_V4/FunctionCall_CANA_send/SEND_line_current ==
  CAN_msg : Inport
  Enable : EnablePort
  CAN_send_line_current : c280xlib/eCAN Transmit  chipFamily=C280x  useModule=eCAN_A  mailboxNo=18  messageID=ID_SEND_LINE_CURRENT  messageType=Standard (11-bit identifier)  enableBlockingMode=off  postInterrupt=off  interruptLine=0
      settings: SourceProductName=Embedded Coder Support Package for Texas Instruments C2000 Processors  SourceProductBaseCode=TIC2000
  wires:
  CAN_msg/1 -> CAN_send_line_current/1

== system BMS_V4/FunctionCall_CANA_send/SEND_send_pso_parameter ==
  CAN_msg : Inport
  Enable : EnablePort
  CAN_send_pso_parameter : c280xlib/eCAN Transmit  chipFamily=C280x  useModule=eCAN_A  mailboxNo=30  messageID=ID_PSO_DEBUG  messageType=Standard (11-bit identifier)  enableBlockingMode=off  postInterrupt=off  interruptLine=0
      settings: SourceProductName=Embedded Coder Support Package for Texas Instruments C2000 Processors  SourceProductBaseCode=TIC2000
  wires:
  CAN_msg/1 -> CAN_send_pso_parameter/1

== system BMS_V4/FunctionCall_CANA_send/SEND_send_system_debug ==
  CAN_msg : Inport
  Enable : EnablePort
  CAN_send_system_debug : c280xlib/eCAN Transmit  chipFamily=C280x  useModule=eCAN_A  mailboxNo=26  messageID=ID_SYSTEM_DEBUG  messageType=Standard (11-bit identifier)  enableBlockingMode=off  postInterrupt=off  interruptLine=0
      settings: SourceProductName=Embedded Coder Support Package for Texas Instruments C2000 Processors  SourceProductBaseCode=TIC2000
  wires:
  CAN_msg/1 -> CAN_send_system_debug/1

== system BMS_V4/FunctionCall_CANA_send/SEND_warning ==
  CAN_msg : Inport
  Enable : EnablePort
  CAN_send_warning : c280xlib/eCAN Transmit  chipFamily=C280x  useModule=eCAN_A  mailboxNo=31  messageID=ID_SEND_WARNING  messageType=Standard (11-bit identifier)  enableBlockingMode=off  postInterrupt=off  interruptLine=0
      settings: SourceProductName=Embedded Coder Support Package for Texas Instruments C2000 Processors  SourceProductBaseCode=TIC2000
  wires:
  CAN_msg/1 -> CAN_send_warning/1

== system BMS_V4/FunctionCall_CANB_RX/handle_active_balance ==
  CAN_msg : Inport
  handle_balance : TriggerPort  TriggerType=function-call  VariantControl=Variant
  balance_proceeding : MATLAB Function  TreatAsAtomicUnit=on
      settings: RTWSystemCode=Nonreusable function  RTWFcnNameOpts=Use subsystem name  RTWFileNameOpts=Use subsystem name
  wires:
  CAN_msg/1 -> balance_proceeding/1(msg)

== system BMS_V4/FunctionCall_CANB_RX/handle_balance ==
  CAN_msg : Inport
  handle_balance : TriggerPort  TriggerType=function-call  VariantControl=Variant
  balance_proceeding : MATLAB Function  TreatAsAtomicUnit=on
      settings: RTWSystemCode=Nonreusable function  RTWFcnNameOpts=Use subsystem name  RTWFileNameOpts=Use subsystem name
  wires:
  CAN_msg/1 -> balance_proceeding/1(msg)

== system BMS_V4/FunctionCall_CANB_RX/handle_cellT_burst ==
  CAN_msg : Inport
  handle_cellT_burst : TriggerPort  TriggerType=function-call  VariantControl=Variant
  cellT_proceeding : MATLAB Function  TreatAsAtomicUnit=on
      settings: RTWSystemCode=Nonreusable function  RTWFcnNameOpts=Use subsystem name  RTWFileNameOpts=Use subsystem name
  wires:
  CAN_msg/1 -> cellT_proceeding/1(msg)

== system BMS_V4/FunctionCall_CANB_RX/handle_cellV_burst ==
  CAN_msg : Inport
  handle_cellV_burst : TriggerPort  TriggerType=function-call  VariantControl=Variant
  cellV_proceeding : MATLAB Function  TreatAsAtomicUnit=on
      settings: RTWSystemCode=Nonreusable function  RTWFcnNameOpts=Use subsystem name  RTWFileNameOpts=Use subsystem name  FunctionInterfaceSpec=Allow arguments
  wires:
  CAN_msg/1 -> cellV_proceeding/1(msg)

== system BMS_V4/FunctionCall_CANB_RX/handle_contactor ==
  CAN_msg : Inport
  handle_contactor : TriggerPort  TriggerType=function-call  VariantControl=Variant
  contactor_proceeding : MATLAB Function  TreatAsAtomicUnit=on
      settings: RTWSystemCode=Nonreusable function  RTWFcnNameOpts=Use subsystem name  RTWFileNameOpts=Use subsystem name
  wires:
  CAN_msg/1 -> contactor_proceeding/1(msg)

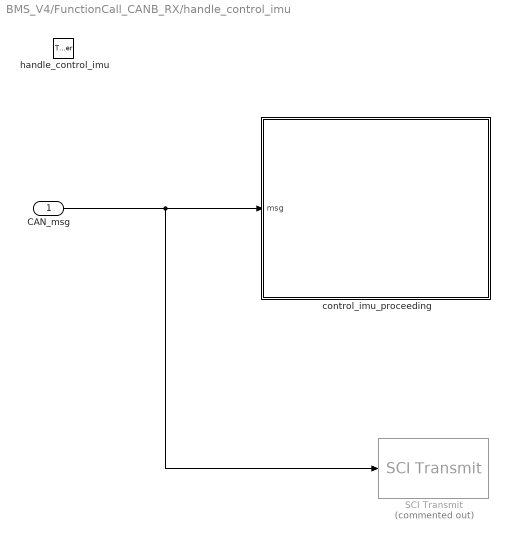
== system BMS_V4/FunctionCall_CANB_RX/handle_control_imu ==
  CAN_msg : Inport
  handle_control_imu : TriggerPort  TriggerType=function-call  VariantControl=Variant
  SCI Transmit : c280xlib/SCI Transmit  Commented=on  sciModule=B  dataHead='S'  dataTail='E'  postInterrupt=off  numFifo=1
      settings: SourceProductName=Embedded Coder Support Package for Texas Instruments C2000 Processors
  control_imu_proceeding : MATLAB Function  TreatAsAtomicUnit=on
      settings: RTWSystemCode=Nonreusable function  RTWFcnNameOpts=Use subsystem name  RTWFileNameOpts=Use subsystem name
  wires:
  CAN_msg/1 -> SCI Transmit/1, control_imu_proceeding/1(msg)

== system BMS_V4/FunctionCall_CANB_RX/handle_info ==
  CAN_msg : Inport
  handle_info : TriggerPort  TriggerType=function-call  VariantControl=Variant
  info_proceeding : MATLAB Function  TreatAsAtomicUnit=on
      settings: RTWSystemCode=Nonreusable function  RTWFcnNameOpts=Use subsystem name  RTWFileNameOpts=Use subsystem name
  wires:
  CAN_msg/1 -> info_proceeding/1(msg)

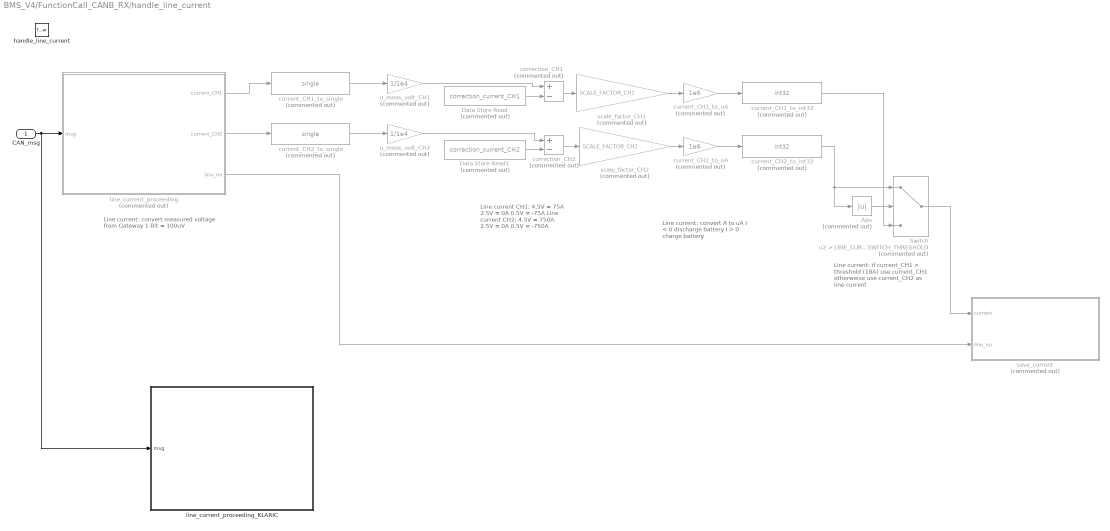
== system BMS_V4/FunctionCall_CANB_RX/handle_line_current ==
  note: Line current:
      | if current_CH1 > threshold (18A)
      | use current_CH1 otherweise
      | use current_CH2 as line current
  note: Line current:
      | convert A to uA
      | I < 0 discharge battery
      | I > 0 charge battery
  note: Line current CH1:
      | 4.5V = 75A
      | 2.5V = 0A
      | 0.5V = -75A
      | Line current CH2:
      | 4.5V = 750A
      | 2.5V = 0A
      | 0.5V = -750A
  note: Line current:
      | convert measured voltage from Gateway
      | 1 Bit = 100uV
  CAN_msg : Inport
  handle_line_current : TriggerPort  TriggerType=function-call  VariantControl=Variant
  Abs : Abs  Commented=on
  Data Store Read : DataStoreRead  Commented=on  DataStoreName=correction_current_CH1
  Data Store Read1 : DataStoreRead  Commented=on  DataStoreName=correction_current_CH2
  Switch : Switch  Commented=on  Criteria=u2 > Threshold  Threshold=LINE_CURRENT_SWITCH_THRESHOLD  OutDataTypeStr=int32
  correction_CH1 : Sum  Commented=on  Inputs=+-
  correction_CH2 : Sum  Commented=on  Inputs=+-
  current_CH1_to_int32 : DataTypeConversion  Commented=on  OutDataTypeStr=int32
  current_CH1_to_single : DataTypeConversion  Commented=on  OutDataTypeStr=single
  current_CH1_to_uA : Gain  Commented=on  Gain=1e6
  current_CH2_to_int32 : DataTypeConversion  Commented=on  OutDataTypeStr=int32
  current_CH2_to_single : DataTypeConversion  Commented=on  OutDataTypeStr=single
  current_CH2_to_uA : Gain  Commented=on  Gain=1e6
  line_current_proceeding : MATLAB Function  Commented=on  TreatAsAtomicUnit=on
      settings: RTWSystemCode=Nonreusable function  RTWFcnNameOpts=Use subsystem name  RTWFileNameOpts=Use subsystem name
  line_current_proceeding_KLARIC : MATLAB Function  TreatAsAtomicUnit=on
      settings: RTWSystemCode=Nonreusable function  RTWFcnNameOpts=Use subsystem name  RTWFileNameOpts=Use subsystem name
  save_current : MATLAB Function  Commented=on  TreatAsAtomicUnit=on
      settings: RTWSystemCode=Nonreusable function  RTWFcnNameOpts=Use subsystem name  RTWFileNameOpts=Use subsystem name
  scale_factor_CH1 : Gain  Commented=on  Gain=SCALE_FACTOR_CH1
  scale_factor_CH2 : Gain  Commented=on  Gain=SCALE_FACTOR_CH2
  u_meas_volt_CH1 : Gain  Commented=on  Gain=1/1e4
  u_meas_volt_CH2 : Gain  Commented=on  Gain=1/1e4
  wires:
  CAN_msg/1 -> line_current_proceeding/1(msg), line_current_proceeding_KLARIC/1(msg)
  line_current_proceeding/1(current_CH1) -> current_CH1_to_single/1
  current_CH1_to_uA/1 -> current_CH1_to_int32/1
  current_CH2_to_uA/1 -> current_CH2_to_int32/1
  Abs/1 -> Switch/2
  line_current_proceeding/3(line_no) -> save_current/2(line_no)
  line_current_proceeding/2(current_CH2) -> current_CH2_to_single/1
  u_meas_volt_CH1/1 -> correction_CH1/1
  correction_CH1/1 -> scale_factor_CH1/1
  Data Store Read/1 -> correction_CH1/2
  current_CH1_to_single/1 -> u_meas_volt_CH1/1
  scale_factor_CH1/1 -> current_CH1_to_uA/1
  current_CH2_to_single/1 -> u_meas_volt_CH2/1
  Data Store Read1/1 -> correction_CH2/2
  u_meas_volt_CH2/1 -> correction_CH2/1
  correction_CH2/1 -> scale_factor_CH2/1
  scale_factor_CH2/1 -> current_CH2_to_uA/1
  current_CH2_to_int32/1 -> Switch/1, Abs/1
  Switch/1 -> save_current/1(current)
  current_CH1_to_int32/1 -> Switch/3

== system BMS_V4/FunctionCalll_CANB_send/INIT_active_balance ==
  CAN_msg : Inport
  Enable : EnablePort
  init_balance : c280xlib/eCAN Transmit  chipFamily=C280x  useModule=eCAN_B  mailboxNo=0  messageID=ID_INIT_ACTIVE_BALANCE  messageType=Standard (11-bit identifier)  enableBlockingMode=off  postInterrupt=off  interruptLine=0
      settings: SourceProductName=Embedded Coder Support Package for Texas Instruments C2000 Processors  SourceProductBaseCode=TIC2000
  wires:
  CAN_msg/1 -> init_balance/1

== system BMS_V4/FunctionCalll_CANB_send/INIT_balance ==
  CAN_msg : Inport
  Enable : EnablePort
  init_balance : c280xlib/eCAN Transmit  chipFamily=C280x  useModule=eCAN_B  mailboxNo=4  messageID=ID_INIT_BALANCE  messageType=Standard (11-bit identifier)  enableBlockingMode=off  postInterrupt=off  interruptLine=0
      settings: SourceProductName=Embedded Coder Support Package for Texas Instruments C2000 Processors  SourceProductBaseCode=TIC2000
  wires:
  CAN_msg/1 -> init_balance/1

== system BMS_V4/FunctionCalll_CANB_send/INIT_cellT_burst ==
  CAN_msg : Inport
  Enable : EnablePort
  init_cellT_burst : c280xlib/eCAN Transmit  chipFamily=C280x  useModule=eCAN_B  mailboxNo=2  messageID=ID_INIT_CELLT_BURST  messageType=Standard (11-bit identifier)  enableBlockingMode=off  postInterrupt=off  interruptLine=0
      settings: SourceProductName=Embedded Coder Support Package for Texas Instruments C2000 Processors  SourceProductBaseCode=TIC2000
  wires:
  CAN_msg/1 -> init_cellT_burst/1

== system BMS_V4/FunctionCalll_CANB_send/INIT_cellV_burst ==
  CAN_msg : Inport
  Enable : EnablePort
  init_cellV_burst : c280xlib/eCAN Transmit  chipFamily=C280x  useModule=eCAN_B  mailboxNo=1  messageID=ID_INIT_CELLV_BURST  messageType=Standard (11-bit identifier)  enableBlockingMode=off  postInterrupt=off  interruptLine=0
      settings: SourceProductName=Embedded Coder Support Package for Texas Instruments C2000 Processors  SourceProductBaseCode=TIC2000
  wires:
  CAN_msg/1 -> init_cellV_burst/1

== system BMS_V4/FunctionCalll_CANB_send/INIT_contactor ==
  CAN_msg : Inport
  Enable : EnablePort
  init_contactor : c280xlib/eCAN Transmit  chipFamily=C280x  useModule=eCAN_B  mailboxNo=6  messageID=ID_INIT_CONTACTOR  messageType=Standard (11-bit identifier)  enableBlockingMode=off  postInterrupt=off  interruptLine=0
      settings: SourceProductName=Embedded Coder Support Package for Texas Instruments C2000 Processors  SourceProductBaseCode=TIC2000
  wires:
  CAN_msg/1 -> init_contactor/1

== system BMS_V4/FunctionCalll_CANB_send/INIT_control_imu ==
  CAN_msg : Inport
  Enable : EnablePort
  init_control_imu : c280xlib/eCAN Transmit  chipFamily=C280x  useModule=eCAN_B  mailboxNo=13  messageID=ID_INIT_CONTROL_IMU  messageType=Standard (11-bit identifier)  enableBlockingMode=off  postInterrupt=off  interruptLine=0
      settings: SourceProductName=Embedded Coder Support Package for Texas Instruments C2000 Processors  SourceProductBaseCode=TIC2000
  wires:
  CAN_msg/1 -> init_control_imu/1

== system BMS_V4/FunctionCalll_CANB_send/INIT_info ==
  CAN_msg : Inport
  Enable : EnablePort
  init_info : c280xlib/eCAN Transmit  chipFamily=C280x  useModule=eCAN_B  mailboxNo=5  messageID=ID_INIT_INFO  messageType=Standard (11-bit identifier)  enableBlockingMode=off  postInterrupt=off  interruptLine=0
      settings: SourceProductName=Embedded Coder Support Package for Texas Instruments C2000 Processors  SourceProductBaseCode=TIC2000
  wires:
  CAN_msg/1 -> init_info/1

== system BMS_V4/FunctionCalll_CANB_send/INIT_line_current ==
  CAN_msg : Inport
  Enable : EnablePort
  init_line_current : c280xlib/eCAN Transmit  chipFamily=C280x  useModule=eCAN_B  mailboxNo=3  messageID=ID_INIT_LINE_CURRENT  messageType=Standard (11-bit identifier)  enableBlockingMode=off  postInterrupt=off  interruptLine=0
      settings: SourceProductName=Embedded Coder Support Package for Texas Instruments C2000 Processors  SourceProductBaseCode=TIC2000
  wires:
  CAN_msg/1 -> init_line_current/1

== system BMS_V4/timer_init/System Initialize ==
